simulink model "main_SEPETC"  (R2021a)
settings: Solver=VariableStepAuto  StartTime=0.0  StopTime=10  RelTol=1e-3
InitFcn:
  | run('Parameter.m')
values from neighbouring files (symbols this model uses):
  cp = 1    [Parameter.m]
  cv = 5    [Parameter.m]
  cw = 5    [Parameter.m]
  fref = 60    [Parameter.m]
  Lc1 = 0.35e-3    (= 0.00035)    [Parameter.m]
  Lc2 = 0.35e-3    (= 0.00035)    [Parameter.m]
  Lc3 = 0.35e-3    (= 0.00035)    [Parameter.m]
  Lc4 = 0.35e-3    (= 0.00035)    [Parameter.m]
  Lt12 = 318e-6    (= 0.000318)    [Parameter.m]
  Lt23 = 1847e-6    (= 0.001847)    [Parameter.m]
  Lt34 = 318e-6    (= 0.000318)    [Parameter.m]
  Mp1 = 9.4e-5    (= 9.4e-05)    [Parameter.m]
  Mp2 = 9.4e-5    (= 9.4e-05)    [Parameter.m]
  Mp3 = 12.5e-5    (= 0.000125)    [Parameter.m]
  Mp4 = 12.5e-5    (= 0.000125)    [Parameter.m]
  Nq1 = 1.3e-3    (= 0.0013)    [Parameter.m]
  Nq2 = 1.3e-3    (= 0.0013)    [Parameter.m]
  Nq3 = 1.5e-3    (= 0.0015)    [Parameter.m]
  Nq4 = 1.5e-3    (= 0.0015)    [Parameter.m]
  Rc1 = 0.03    [Parameter.m]
  Rc2 = 0.03    [Parameter.m]
  Rc3 = 0.03    [Parameter.m]
  Rc4 = 0.03    [Parameter.m]
  Rt12 = 0.23    [Parameter.m]
  Rt23 = 0.35    [Parameter.m]
  Rt34 = 0.23    [Parameter.m]
  t2 = 1    [Parameter.m]    (also in wvp_SEPETC.m)
  t3 = 10    [Parameter.m]
  t4 = 20    [Parameter.m]    (also in wvp_SEPETC.m = 21)
  t5 = 35    [Parameter.m]    (also in wvp_SEPETC.m = 33)
  t6 = 40    [Parameter.m]    (also in wvp_SEPETC.m = 35)
  Uo = 220*sqrt(2)    [Parameter.m]
  vref = 380    [Parameter.m]
  wc = 31.4    [Parameter.m]
  wref = 2*pi*fref    (= 376.991118431)    [Parameter.m]
undefined symbols (not defined in the file or in its folder): gcbh, sps_rtmsupport
libraries: spsControlledVoltageSourceLib x12, spsAlphaBetaZerotodq0Lib x12, eeGeneralControl x8, spsThreePhaseSeriesRLCBranchLib x7, spsGroundLib x4, spsThreePhaseVIMeasurementLib x4, spsThreePhaseBreakerLib x4, spsPLL3phLib x4, spsThreePhaseSeriesRLCLoadLib x3, spspowerguiLib x1
(part 3 of 3)

== system main_SEPETC/controller 1/primary 1/(P) abc to dq2 ==
  abc : Inport  PortDimensions=3
  wt : Inport  Port=2  PortDimensions=1
  Alpha-Beta-Zero to dq0 : spsAlphaBetaZerotodq0Lib/Alpha-Beta-Zero to dq0  Alignment=90 degrees behind phase A axis
      settings: SourceProductBaseCode=PS
  abc to Alpha-Beta-Zero : Subsystem  AncestorBlock=powerlib_meascontrol/Transformations/abc to Alpha-Beta-Zero  DialogController=POWERSYS.PowerSysDialog  LoadFcn=sps_rtmsupport('LoadFcn', gcbh);  StartFcn=sps_rtmsupport('StartFcn', gcbh);  StopFcn=sps_rtmsupport('StopFcn', gcbh);  mask(abc to Alpha-Beta-Zero Transformation){}
      mask help: Perform a Clarke transformation from a three-phase (abc) signal to a alpha-beta-zero stationary reference frame.
      settings: CopyFcn=sps_rtmsupport('CopyFcn', gcbh);  DeleteFcn=sps_rtmsupport('DeleteFcn', gcbh);  UndoDeleteFcn=sps_rtmsupport('UndoDeleteFcn', gcbh);  ModelCloseFcn=sps_rtmsupport('ModelCloseFcn', gcbh);  PreSaveFcn=sps_rtmsupport('PreSaveFcn', gcbh);  PostSaveFcn=sps_rtmsupport('PostSaveFcn', gcbh);  NameChangeFcn=sps_rtmsupport('NameChangeFcn', gcbh);  PreCopyFcn=sps_rtmsupport('PreCopyFcn', gcbh);  OpenFcn=sps_rtmsupport('OpenFcn', gcbh, []);  CloseFcn=sps_rtmsupport('CloseFcn', gcbh);  PreDeleteFcn=sps_rtmsupport('PreDeleteFcn', gcbh);
      mask Help: helpview(psbhelp);
      mask Display:
      | plot([0 1], [0,1])
      | text(0.15,0.7,'abc')
      | text(0.55, 0.3,'\alpha\beta0','texmode','on')
  dq0 : Outport  VectorParamsAs1DForOutWhenUnconnected=off
  wires:
  wt/1 -> Alpha-Beta-Zero to dq0/2
  abc/1 -> abc to Alpha-Beta-Zero/1(abc)
  Alpha-Beta-Zero to dq0/1 -> dq0/1
  abc to Alpha-Beta-Zero/1(al_be_0) -> Alpha-Beta-Zero to dq0/1

== system main_SEPETC/controller 2/(P) abc to dq2/abc to Alpha-Beta-Zero ==
  abc : Inport  PortDimensions=3
  Gain1 : Gain  Gain=sqrt(2/3)  SaturateOnIntegerOverflow=on  OutDataTypeStr=Inherit: Same as input  ParamDataTypeStr=Inherit: Same as input
  Gain3 : Gain  Gain="[ 1   -1/2   -1/2; 0   sqrt(3)/2   -sqrt(3)/2; 1/sqrt(2)  1/sqrt(2)  1/sqrt(2) ]"  Multiplication=Matrix(K*u) (u vector)  SaturateOnIntegerOverflow=on  OutDataTypeStr=Inherit: Same as input  ParamDataTypeStr=Inherit: Same as input
  al_be_0 : Outport  VectorParamsAs1DForOutWhenUnconnected=off
  wires:
  abc/1 -> Gain3/1
  Gain3/1 -> Gain1/1
  Gain1/1 -> al_be_0/1

== system main_SEPETC/controller 2/primary 1/(P) abc to dq1 ==
  abc : Inport  PortDimensions=3
  wt : Inport  Port=2  PortDimensions=1
  Alpha-Beta-Zero to dq0 : spsAlphaBetaZerotodq0Lib/Alpha-Beta-Zero to dq0  Alignment=90 degrees behind phase A axis
      settings: SourceProductBaseCode=PS
  abc to Alpha-Beta-Zero : Subsystem  AncestorBlock=powerlib_meascontrol/Transformations/abc to Alpha-Beta-Zero  DialogController=POWERSYS.PowerSysDialog  LoadFcn=sps_rtmsupport('LoadFcn', gcbh);  StartFcn=sps_rtmsupport('StartFcn', gcbh);  StopFcn=sps_rtmsupport('StopFcn', gcbh);  mask(abc to Alpha-Beta-Zero Transformation){}
      mask help: Perform a Clarke transformation from a three-phase (abc) signal to a alpha-beta-zero stationary reference frame.
      settings: CopyFcn=sps_rtmsupport('CopyFcn', gcbh);  DeleteFcn=sps_rtmsupport('DeleteFcn', gcbh);  UndoDeleteFcn=sps_rtmsupport('UndoDeleteFcn', gcbh);  ModelCloseFcn=sps_rtmsupport('ModelCloseFcn', gcbh);  PreSaveFcn=sps_rtmsupport('PreSaveFcn', gcbh);  PostSaveFcn=sps_rtmsupport('PostSaveFcn', gcbh);  NameChangeFcn=sps_rtmsupport('NameChangeFcn', gcbh);  PreCopyFcn=sps_rtmsupport('PreCopyFcn', gcbh);  OpenFcn=sps_rtmsupport('OpenFcn', gcbh, []);  CloseFcn=sps_rtmsupport('CloseFcn', gcbh);  PreDeleteFcn=sps_rtmsupport('PreDeleteFcn', gcbh);
      mask Help: helpview(psbhelp);
      mask Display:
      | plot([0 1], [0,1])
      | text(0.15,0.7,'abc')
      | text(0.55, 0.3,'\alpha\beta0','texmode','on')
  dq0 : Outport  VectorParamsAs1DForOutWhenUnconnected=off
  wires:
  wt/1 -> Alpha-Beta-Zero to dq0/2
  abc/1 -> abc to Alpha-Beta-Zero/1(abc)
  Alpha-Beta-Zero to dq0/1 -> dq0/1
  abc to Alpha-Beta-Zero/1(al_be_0) -> Alpha-Beta-Zero to dq0/1

== system main_SEPETC/controller 2/primary 1/(P) abc to dq2 ==
  abc : Inport  PortDimensions=3
  wt : Inport  Port=2  PortDimensions=1
  Alpha-Beta-Zero to dq0 : spsAlphaBetaZerotodq0Lib/Alpha-Beta-Zero to dq0  Alignment=90 degrees behind phase A axis
      settings: SourceProductBaseCode=PS
  abc to Alpha-Beta-Zero : Subsystem  AncestorBlock=powerlib_meascontrol/Transformations/abc to Alpha-Beta-Zero  DialogController=POWERSYS.PowerSysDialog  LoadFcn=sps_rtmsupport('LoadFcn', gcbh);  StartFcn=sps_rtmsupport('StartFcn', gcbh);  StopFcn=sps_rtmsupport('StopFcn', gcbh);  mask(abc to Alpha-Beta-Zero Transformation){}
      mask help: Perform a Clarke transformation from a three-phase (abc) signal to a alpha-beta-zero stationary reference frame.
      settings: CopyFcn=sps_rtmsupport('CopyFcn', gcbh);  DeleteFcn=sps_rtmsupport('DeleteFcn', gcbh);  UndoDeleteFcn=sps_rtmsupport('UndoDeleteFcn', gcbh);  ModelCloseFcn=sps_rtmsupport('ModelCloseFcn', gcbh);  PreSaveFcn=sps_rtmsupport('PreSaveFcn', gcbh);  PostSaveFcn=sps_rtmsupport('PostSaveFcn', gcbh);  NameChangeFcn=sps_rtmsupport('NameChangeFcn', gcbh);  PreCopyFcn=sps_rtmsupport('PreCopyFcn', gcbh);  OpenFcn=sps_rtmsupport('OpenFcn', gcbh, []);  CloseFcn=sps_rtmsupport('CloseFcn', gcbh);  PreDeleteFcn=sps_rtmsupport('PreDeleteFcn', gcbh);
      mask Help: helpview(psbhelp);
      mask Display:
      | plot([0 1], [0,1])
      | text(0.15,0.7,'abc')
      | text(0.55, 0.3,'\alpha\beta0','texmode','on')
  dq0 : Outport  VectorParamsAs1DForOutWhenUnconnected=off
  wires:
  wt/1 -> Alpha-Beta-Zero to dq0/2
  abc/1 -> abc to Alpha-Beta-Zero/1(abc)
  Alpha-Beta-Zero to dq0/1 -> dq0/1
  abc to Alpha-Beta-Zero/1(al_be_0) -> Alpha-Beta-Zero to dq0/1

== system main_SEPETC/controller 3/(P) abc to dq2/abc to Alpha-Beta-Zero ==
  abc : Inport  PortDimensions=3
  Gain1 : Gain  Gain=sqrt(2/3)  SaturateOnIntegerOverflow=on  OutDataTypeStr=Inherit: Same as input  ParamDataTypeStr=Inherit: Same as input
  Gain3 : Gain  Gain="[ 1   -1/2   -1/2; 0   sqrt(3)/2   -sqrt(3)/2; 1/sqrt(2)  1/sqrt(2)  1/sqrt(2) ]"  Multiplication=Matrix(K*u) (u vector)  SaturateOnIntegerOverflow=on  OutDataTypeStr=Inherit: Same as input  ParamDataTypeStr=Inherit: Same as input
  al_be_0 : Outport  VectorParamsAs1DForOutWhenUnconnected=off
  wires:
  abc/1 -> Gain3/1
  Gain3/1 -> Gain1/1
  Gain1/1 -> al_be_0/1

== system main_SEPETC/controller 3/primary 3/(P) abc to dq1 ==
  abc : Inport  PortDimensions=3
  wt : Inport  Port=2  PortDimensions=1
  Alpha-Beta-Zero to dq0 : spsAlphaBetaZerotodq0Lib/Alpha-Beta-Zero to dq0  Alignment=90 degrees behind phase A axis
      settings: SourceProductBaseCode=PS
  abc to Alpha-Beta-Zero : Subsystem  AncestorBlock=powerlib_meascontrol/Transformations/abc to Alpha-Beta-Zero  DialogController=POWERSYS.PowerSysDialog  LoadFcn=sps_rtmsupport('LoadFcn', gcbh);  StartFcn=sps_rtmsupport('StartFcn', gcbh);  StopFcn=sps_rtmsupport('StopFcn', gcbh);  mask(abc to Alpha-Beta-Zero Transformation){}
      mask help: Perform a Clarke transformation from a three-phase (abc) signal to a alpha-beta-zero stationary reference frame.
      settings: CopyFcn=sps_rtmsupport('CopyFcn', gcbh);  DeleteFcn=sps_rtmsupport('DeleteFcn', gcbh);  UndoDeleteFcn=sps_rtmsupport('UndoDeleteFcn', gcbh);  ModelCloseFcn=sps_rtmsupport('ModelCloseFcn', gcbh);  PreSaveFcn=sps_rtmsupport('PreSaveFcn', gcbh);  PostSaveFcn=sps_rtmsupport('PostSaveFcn', gcbh);  NameChangeFcn=sps_rtmsupport('NameChangeFcn', gcbh);  PreCopyFcn=sps_rtmsupport('PreCopyFcn', gcbh);  OpenFcn=sps_rtmsupport('OpenFcn', gcbh, []);  CloseFcn=sps_rtmsupport('CloseFcn', gcbh);  PreDeleteFcn=sps_rtmsupport('PreDeleteFcn', gcbh);
      mask Help: helpview(psbhelp);
      mask Display:
      | plot([0 1], [0,1])
      | text(0.15,0.7,'abc')
      | text(0.55, 0.3,'\alpha\beta0','texmode','on')
  dq0 : Outport  VectorParamsAs1DForOutWhenUnconnected=off
  wires:
  wt/1 -> Alpha-Beta-Zero to dq0/2
  abc/1 -> abc to Alpha-Beta-Zero/1(abc)
  Alpha-Beta-Zero to dq0/1 -> dq0/1
  abc to Alpha-Beta-Zero/1(al_be_0) -> Alpha-Beta-Zero to dq0/1

== system main_SEPETC/controller 3/primary 3/(P) abc to dq2 ==
  abc : Inport  PortDimensions=3
  wt : Inport  Port=2  PortDimensions=1
  Alpha-Beta-Zero to dq0 : spsAlphaBetaZerotodq0Lib/Alpha-Beta-Zero to dq0  Alignment=90 degrees behind phase A axis
      settings: SourceProductBaseCode=PS
  abc to Alpha-Beta-Zero : Subsystem  AncestorBlock=powerlib_meascontrol/Transformations/abc to Alpha-Beta-Zero  DialogController=POWERSYS.PowerSysDialog  LoadFcn=sps_rtmsupport('LoadFcn', gcbh);  StartFcn=sps_rtmsupport('StartFcn', gcbh);  StopFcn=sps_rtmsupport('StopFcn', gcbh);  mask(abc to Alpha-Beta-Zero Transformation){}
      mask help: Perform a Clarke transformation from a three-phase (abc) signal to a alpha-beta-zero stationary reference frame.
      settings: CopyFcn=sps_rtmsupport('CopyFcn', gcbh);  DeleteFcn=sps_rtmsupport('DeleteFcn', gcbh);  UndoDeleteFcn=sps_rtmsupport('UndoDeleteFcn', gcbh);  ModelCloseFcn=sps_rtmsupport('ModelCloseFcn', gcbh);  PreSaveFcn=sps_rtmsupport('PreSaveFcn', gcbh);  PostSaveFcn=sps_rtmsupport('PostSaveFcn', gcbh);  NameChangeFcn=sps_rtmsupport('NameChangeFcn', gcbh);  PreCopyFcn=sps_rtmsupport('PreCopyFcn', gcbh);  OpenFcn=sps_rtmsupport('OpenFcn', gcbh, []);  CloseFcn=sps_rtmsupport('CloseFcn', gcbh);  PreDeleteFcn=sps_rtmsupport('PreDeleteFcn', gcbh);
      mask Help: helpview(psbhelp);
      mask Display:
      | plot([0 1], [0,1])
      | text(0.15,0.7,'abc')
      | text(0.55, 0.3,'\alpha\beta0','texmode','on')
  dq0 : Outport  VectorParamsAs1DForOutWhenUnconnected=off
  wires:
  wt/1 -> Alpha-Beta-Zero to dq0/2
  abc/1 -> abc to Alpha-Beta-Zero/1(abc)
  Alpha-Beta-Zero to dq0/1 -> dq0/1
  abc to Alpha-Beta-Zero/1(al_be_0) -> Alpha-Beta-Zero to dq0/1

== system main_SEPETC/controller 3/v_secondary 3/Subsystem2 ==
  In1 : Inport
  Constant : Constant  Value=0
  Switch : Switch  Criteria=u2 > Threshold
  Out1 : Outport
  wires:
  [t] -> Switch/2
  Switch/1 -> Out1/1
  Constant/1 -> Switch/3
  In1/1 -> Switch/1

== system main_SEPETC/controller 3/w_secondary 3/Subsystem2 ==
  In1 : Inport
  Constant : Constant  Value=0
  Switch : Switch  Criteria=u2 > Threshold
  Out1 : Outport
  wires:
  [t] -> Switch/2
  Switch/1 -> Out1/1
  Constant/1 -> Switch/3
  In1/1 -> Switch/1

== system main_SEPETC/controller 4/(P) abc to dq2/abc to Alpha-Beta-Zero ==
  abc : Inport  PortDimensions=3
  Gain1 : Gain  Gain=sqrt(2/3)  SaturateOnIntegerOverflow=on  OutDataTypeStr=Inherit: Same as input  ParamDataTypeStr=Inherit: Same as input
  Gain3 : Gain  Gain="[ 1   -1/2   -1/2; 0   sqrt(3)/2   -sqrt(3)/2; 1/sqrt(2)  1/sqrt(2)  1/sqrt(2) ]"  Multiplication=Matrix(K*u) (u vector)  SaturateOnIntegerOverflow=on  OutDataTypeStr=Inherit: Same as input  ParamDataTypeStr=Inherit: Same as input
  al_be_0 : Outport  VectorParamsAs1DForOutWhenUnconnected=off
  wires:
  abc/1 -> Gain3/1
  Gain3/1 -> Gain1/1
  Gain1/1 -> al_be_0/1

== system main_SEPETC/controller 4/primary 3/Subsystem1 ==
  note: D-Q变换
  Vo1 : Inport
  wt : Inport  Port=2
  io1 : Inport  Port=3
  (P) abc to dq1 : Subsystem  AncestorBlock=powerlib_meascontrol/Transformations/abc to dq0  DialogController=POWERSYS.PowerSysDialog  LoadFcn=sps_rtmsupport('LoadFcn', gcbh);  StartFcn=sps_rtmsupport('StartFcn', gcbh);  StopFcn=sps_rtmsupport('StopFcn', gcbh);  mask(abc to dq0 Transformation){Alignment=90 degrees behind phase A axis}
      mask prompts: Alignment "Rotating frame alignment at wt=0:"
      mask help:
      | Perform a Park transformation from a three-phase (abc) signal to a dq0 rotating reference frame. Angular position of the rotating frame is given by input wt (rad).
      |
      | When the rotating frame alignment at wt=0 is 90 degrees behind phase A axis, a positive-sequence signal with Mag=1 & Phase=0 degrees yields the following dq values: d=1, q=0.
      mask init:
      | str=cat(2,gcb,'/Alpha-Beta-Zero to dq0');
      | if Alignment==1
      |     set_param(str,'Alignment','Aligned with phase A axis');
      | else
      |     set_param(str,'Alignment','90 degrees behind phase A axis');
      | end
      settings: CopyFcn=sps_rtmsupport('CopyFcn', gcbh);  DeleteFcn=sps_rtmsupport('DeleteFcn', gcbh);  UndoDeleteFcn=sps_rtmsupport('UndoDeleteFcn', gcbh);  ModelCloseFcn=sps_rtmsupport('ModelCloseFcn', gcbh);  PreSaveFcn=sps_rtmsupport('PreSaveFcn', gcbh);  PostSaveFcn=sps_rtmsupport('PostSaveFcn', gcbh);  NameChangeFcn=sps_rtmsupport('NameChangeFcn', gcbh);  PreCopyFcn=sps_rtmsupport('PreCopyFcn', gcbh);  OpenFcn=sps_rtmsupport('OpenFcn', gcbh, [1]);  CloseFcn=sps_rtmsupport('CloseFcn', gcbh);  PreDeleteFcn=sps_rtmsupport('PreDeleteFcn', gcbh);
      mask Help: helpview(psbhelp);
      mask TypeOptions Alignment: Aligned with phase A axis | 90 degrees behind phase A axis
      mask Display:
      | plot([0 1], [0,1])
      | port_label('input', 1, 'abc')
      | port_label('input', 2, 'wt')
      | port_label('output', 1, 'dq0')
  (P) abc to dq2 : Subsystem  AncestorBlock=powerlib_meascontrol/Transformations/abc to dq0  DialogController=POWERSYS.PowerSysDialog  LoadFcn=sps_rtmsupport('LoadFcn', gcbh);  StartFcn=sps_rtmsupport('StartFcn', gcbh);  StopFcn=sps_rtmsupport('StopFcn', gcbh);  mask(abc to dq0 Transformation){Alignment=90 degrees behind phase A axis}
      mask prompts: Alignment "Rotating frame alignment at wt=0:"
      mask help:
      | Perform a Park transformation from a three-phase (abc) signal to a dq0 rotating reference frame. Angular position of the rotating frame is given by input wt (rad).
      |
      | When the rotating frame alignment at wt=0 is 90 degrees behind phase A axis, a positive-sequence signal with Mag=1 & Phase=0 degrees yields the following dq values: d=1, q=0.
      mask init:
      | str=cat(2,gcb,'/Alpha-Beta-Zero to dq0');
      | if Alignment==1
      |     set_param(str,'Alignment','Aligned with phase A axis');
      | else
      |     set_param(str,'Alignment','90 degrees behind phase A axis');
      | end
      settings: CopyFcn=sps_rtmsupport('CopyFcn', gcbh);  DeleteFcn=sps_rtmsupport('DeleteFcn', gcbh);  UndoDeleteFcn=sps_rtmsupport('UndoDeleteFcn', gcbh);  ModelCloseFcn=sps_rtmsupport('ModelCloseFcn', gcbh);  PreSaveFcn=sps_rtmsupport('PreSaveFcn', gcbh);  PostSaveFcn=sps_rtmsupport('PostSaveFcn', gcbh);  NameChangeFcn=sps_rtmsupport('NameChangeFcn', gcbh);  PreCopyFcn=sps_rtmsupport('PreCopyFcn', gcbh);  OpenFcn=sps_rtmsupport('OpenFcn', gcbh, [1]);  CloseFcn=sps_rtmsupport('CloseFcn', gcbh);  PreDeleteFcn=sps_rtmsupport('PreDeleteFcn', gcbh);
      mask Help: helpview(psbhelp);
      mask TypeOptions Alignment: Aligned with phase A axis | 90 degrees behind phase A axis
      mask Display:
      | plot([0 1], [0,1])
      | port_label('input', 1, 'abc')
      | port_label('input', 2, 'wt')
      | port_label('output', 1, 'dq0')
  Demux : Demux  Outputs=2
  Demux1 : Demux  Outputs=2
  Gain : Gain
  Gain1 : Gain
  Product{,1..3} (4 alike) : Product
  Selector : Selector  InputPortWidth=3  IndexOptions=Index vector (dialog)  Indices=[1 2]  OutputSizes=1
  Selector1 : Selector  InputPortWidth=3  IndexOptions=Index vector (dialog)  Indices=[1 2]  OutputSizes=1
  Sum2 : Sum  Inputs=|++
  Sum3 : Sum  Inputs=|-+
  p' : Outport
  q' : Outport  Port=2
  wires:
  Selector/1 -> Demux/1
  Demux/2 -> Product1/1, Product3/1  "voqi"
  Selector1/1 -> Demux1/1
  wt/1 -> (P) abc to dq1/2(wt), (P) abc to dq2/2(wt)
  Demux/1 -> Product2/1, Product/1  "vodi"
  (P) abc to dq2/1(dq0) -> Selector/1
  Demux1/1 -> Product3/2, Product/2  "iodi"
  (P) abc to dq1/1(dq0) -> Selector1/1
  Product3/1 -> Sum3/2
  Product2/1 -> Sum3/1
  Demux1/2 -> Product1/2, Product2/2  "ioqi"
  Product1/1 -> Sum2/2
  Product/1 -> Sum2/1
  io1/1 -> (P) abc to dq1/1(abc)
  Vo1/1 -> (P) abc to dq2/1(abc)
  Sum2/1 -> Gain/1
  Sum3/1 -> Gain1/1
  Gain1/1 -> q'/1
  Gain/1 -> p'/1

== system main_SEPETC/active power sharing SE-PETC /EState_1/x1_o2/Subsystem1 ==
  In1 : Inport
  Constant : Constant  Value=0
  Switch : Switch  Criteria=u2 > Threshold
  Out1 : Outport
  wires:
  [t] -> Switch/2
  Switch/1 -> Out1/1
  Constant/1 -> Switch/3
  In1/1 -> Switch/1

== system main_SEPETC/active power sharing SE-PETC /EState_1/x1_o4/Subsystem4 ==
  In1 : Inport
  Constant : Constant  Value=0
  Switch : Switch  Criteria=u2 > Threshold
  Out1 : Outport
  wires:
  [t] -> Switch/2
  Switch/1 -> Out1/1
  Constant/1 -> Switch/3
  In1/1 -> Switch/1

== system main_SEPETC/active power sharing SE-PETC /EState_2/x2_o2/Subsystem1 ==
  In1 : Inport
  Constant : Constant  Value=0
  Switch : Switch  Criteria=u2 > Threshold
  Out1 : Outport
  wires:
  [t] -> Switch/2
  Switch/1 -> Out1/1
  In1/1 -> Switch/1
  Constant/1 -> Switch/3

== system main_SEPETC/active power sharing SE-PETC /EState_2/x2_o3/Subsystem1 ==
  In1 : Inport
  Constant : Constant  Value=0
  Switch : Switch  Criteria=u2 > Threshold
  Out1 : Outport
  wires:
  [t] -> Switch/2
  Switch/1 -> Out1/1
  Constant/1 -> Switch/3
  In1/1 -> Switch/1

== system main_SEPETC/active power sharing SE-PETC /EState_2/x2_o3/Subsystem2 ==
  In1 : Inport
  Constant : Constant  Value=0
  Switch : Switch  Criteria=u2 > Threshold
  Out1 : Outport
  wires:
  [t] -> Switch/2
  Switch/1 -> Out1/1
  Constant/1 -> Switch/3
  In1/1 -> Switch/1

== system main_SEPETC/active power sharing SE-PETC /EState_2/x2_o3/Subsystem3 ==
  In1 : Inport
  Constant : Constant  Value=0
  Switch : Switch  Criteria=u2 > Threshold
  Out1 : Outport
  wires:
  [t] -> Switch/2
  Switch/1 -> Out1/1
  Constant/1 -> Switch/3
  In1/1 -> Switch/1

== system main_SEPETC/active power sharing SE-PETC /EState_2/x2_o3/Subsystem4 ==
  In1 : Inport
  Constant : Constant  Value=0
  Switch : Switch  Criteria=u2 > Threshold
  Out1 : Outport
  wires:
  [t] -> Switch/2
  Switch/1 -> Out1/1
  Constant/1 -> Switch/3
  In1/1 -> Switch/1

== system main_SEPETC/active power sharing SE-PETC /EState_3/x3_o2/Subsystem1 ==
  In1 : Inport
  Constant : Constant  Value=0
  Switch : Switch  Criteria=u2 > Threshold
  Out1 : Outport
  wires:
  [t] -> Switch/2
  Switch/1 -> Out1/1
  Constant/1 -> Switch/3
  In1/1 -> Switch/1

== system main_SEPETC/active power sharing SE-PETC /EState_3/x3_o2/Subsystem2 ==
  In1 : Inport
  Constant : Constant  Value=0
  Switch : Switch  Criteria=u2 > Threshold
  Out1 : Outport
  wires:
  [t] -> Switch/2
  Switch/1 -> Out1/1
  Constant/1 -> Switch/3
  In1/1 -> Switch/1

== system main_SEPETC/active power sharing SE-PETC /EState_3/x3_o2/Subsystem3 ==
  In1 : Inport
  Constant : Constant  Value=0
  Switch : Switch  Criteria=u2 > Threshold
  Out1 : Outport
  wires:
  [t] -> Switch/2
  Switch/1 -> Out1/1
  Constant/1 -> Switch/3
  In1/1 -> Switch/1

== system main_SEPETC/active power sharing SE-PETC /EState_3/x3_o2/Subsystem4 ==
  In1 : Inport
  Constant : Constant  Value=0
  Switch : Switch  Criteria=u2 > Threshold
  Out1 : Outport
  wires:
  [t] -> Switch/2
  Switch/1 -> Out1/1
  Constant/1 -> Switch/3
  In1/1 -> Switch/1

== system main_SEPETC/active power sharing SE-PETC /EState_3/x3_o3/Subsystem1 ==
  In1 : Inport
  Constant : Constant  Value=0
  Switch : Switch  Criteria=u2 > Threshold
  Out1 : Outport
  wires:
  [t] -> Switch/2
  Switch/1 -> Out1/1
  Constant/1 -> Switch/3
  In1/1 -> Switch/1

== system main_SEPETC/active power sharing SE-PETC /EState_3/x3_o3/Subsystem2 ==
  In1 : Inport
  Constant : Constant  Value=0
  Switch : Switch  Criteria=u2 > Threshold
  Out1 : Outport
  wires:
  [t] -> Switch/2
  Switch/1 -> Out1/1
  Constant/1 -> Switch/3
  In1/1 -> Switch/1

== system main_SEPETC/active power sharing SE-PETC /EState_3/x3_o3/Subsystem3 ==
  In1 : Inport
  Constant : Constant  Value=0
  Switch : Switch  Criteria=u2 > Threshold
  Out1 : Outport
  wires:
  [t] -> Switch/2
  Switch/1 -> Out1/1
  Constant/1 -> Switch/3
  In1/1 -> Switch/1

== system main_SEPETC/active power sharing SE-PETC /EState_3/x3_o3/Subsystem4 ==
  In1 : Inport
  Constant : Constant  Value=0
  Switch : Switch  Criteria=u2 > Threshold
  Out1 : Outport
  wires:
  [t] -> Switch/2
  Switch/1 -> Out1/1
  Constant/1 -> Switch/3
  In1/1 -> Switch/1

== system main_SEPETC/active power sharing SE-PETC /EState_3/x3_o4/Subsystem1 ==
  In1 : Inport
  Constant : Constant  Value=0
  Switch : Switch  Criteria=u2 > Threshold
  Out1 : Outport
  wires:
  [t] -> Switch/2
  Switch/1 -> Out1/1
  Constant/1 -> Switch/3
  In1/1 -> Switch/1

== system main_SEPETC/active power sharing SE-PETC /EState_3/x3_o4/Subsystem2 ==
  In1 : Inport
  Constant : Constant  Value=0
  Switch : Switch  Criteria=u2 > Threshold
  Out1 : Outport
  wires:
  [t] -> Switch/2
  Switch/1 -> Out1/1
  Constant/1 -> Switch/3
  In1/1 -> Switch/1

== system main_SEPETC/active power sharing SE-PETC /EState_3/x3_o4/Subsystem3 ==
  In1 : Inport
  Constant : Constant  Value=0
  Switch : Switch  Criteria=u2 > Threshold
  Out1 : Outport
  wires:
  [t] -> Switch/2
  Switch/1 -> Out1/1
  Constant/1 -> Switch/3
  In1/1 -> Switch/1

== system main_SEPETC/active power sharing SE-PETC /EState_3/x3_o4/Subsystem4 ==
  In1 : Inport
  Constant : Constant  Value=0
  Switch : Switch  Criteria=u2 > Threshold
  x3_o4 : Outport
  wires:
  [t] -> Switch/2
  Switch/1 -> x3_o4/1
  Constant/1 -> Switch/3
  In1/1 -> Switch/1

== system main_SEPETC/active power sharing SE-PETC /EState_4/x4_o3/Subsystem1 ==
  In1 : Inport
  Constant : Constant  Value=0
  Switch : Switch  Criteria=u2 > Threshold
  Out1 : Outport
  wires:
  [t] -> Switch/2
  Switch/1 -> Out1/1
  Constant/1 -> Switch/3
  In1/1 -> Switch/1

== system main_SEPETC/active power sharing SE-PETC /EState_4/x4_o3/Subsystem2 ==
  In1 : Inport
  Constant : Constant  Value=0
  Switch : Switch  Criteria=u2 > Threshold
  Out1 : Outport
  wires:
  [t] -> Switch/2
  Switch/1 -> Out1/1
  Constant/1 -> Switch/3
  In1/1 -> Switch/1

== system main_SEPETC/active power sharing SE-PETC /EState_4/x4_o3/Subsystem3 ==
  In1 : Inport
  Constant : Constant  Value=0
  Switch : Switch  Criteria=u2 > Threshold
  Out1 : Outport
  wires:
  [t] -> Switch/2
  Switch/1 -> Out1/1
  Constant/1 -> Switch/3
  In1/1 -> Switch/1

== system main_SEPETC/active power sharing SE-PETC /EState_4/x4_o3/Subsystem4 ==
  In1 : Inport
  Constant : Constant  Value=0
  Switch : Switch  Criteria=u2 > Threshold
  Out1 : Outport
  wires:
  [t] -> Switch/2
  Switch/1 -> Out1/1
  Constant/1 -> Switch/3
  In1/1 -> Switch/1

== system main_SEPETC/active power sharing SE-PETC /EState_4/x4_o4/Subsystem1 ==
  In1 : Inport
  Constant : Constant  Value=0
  Switch : Switch  Criteria=u2 > Threshold
  Out1 : Outport
  wires:
  [t] -> Switch/2
  Switch/1 -> Out1/1
  Constant/1 -> Switch/3
  In1/1 -> Switch/1

== system main_SEPETC/active power sharing SE-PETC 1/EState_1/x1_o2/Subsystem1 ==
  In1 : Inport
  Constant : Constant  Value=0
  Switch : Switch  Criteria=u2 > Threshold
  Out1 : Outport
  wires:
  [t] -> Switch/2
  Switch/1 -> Out1/1
  Constant/1 -> Switch/3
  In1/1 -> Switch/1

== system main_SEPETC/active power sharing SE-PETC 1/EState_1/x1_o4/Subsystem4 ==
  In1 : Inport
  Constant : Constant  Value=0
  Switch : Switch  Criteria=u2 > Threshold
  Out1 : Outport
  wires:
  [t] -> Switch/2
  Switch/1 -> Out1/1
  Constant/1 -> Switch/3
  In1/1 -> Switch/1

== system main_SEPETC/active power sharing SE-PETC 1/EState_2/x2_o2/Subsystem1 ==
  In1 : Inport
  Constant : Constant  Value=0
  Switch : Switch  Criteria=u2 > Threshold
  Out1 : Outport
  wires:
  [t] -> Switch/2
  Switch/1 -> Out1/1
  In1/1 -> Switch/1
  Constant/1 -> Switch/3

== system main_SEPETC/active power sharing SE-PETC 1/EState_2/x2_o3/Subsystem1 ==
  In1 : Inport
  Constant : Constant  Value=0
  Switch : Switch  Criteria=u2 > Threshold
  Out1 : Outport
  wires:
  [t] -> Switch/2
  Switch/1 -> Out1/1
  Constant/1 -> Switch/3
  In1/1 -> Switch/1

== system main_SEPETC/active power sharing SE-PETC 1/EState_2/x2_o3/Subsystem2 ==
  In1 : Inport
  Constant : Constant  Value=0
  Switch : Switch  Criteria=u2 > Threshold
  Out1 : Outport
  wires:
  [t] -> Switch/2
  Switch/1 -> Out1/1
  Constant/1 -> Switch/3
  In1/1 -> Switch/1

== system main_SEPETC/active power sharing SE-PETC 1/EState_2/x2_o3/Subsystem3 ==
  In1 : Inport
  Constant : Constant  Value=0
  Switch : Switch  Criteria=u2 > Threshold
  Out1 : Outport
  wires:
  [t] -> Switch/2
  Switch/1 -> Out1/1
  Constant/1 -> Switch/3
  In1/1 -> Switch/1

== system main_SEPETC/active power sharing SE-PETC 1/EState_2/x2_o3/Subsystem4 ==
  In1 : Inport
  Constant : Constant  Value=0
  Switch : Switch  Criteria=u2 > Threshold
  Out1 : Outport
  wires:
  [t] -> Switch/2
  Switch/1 -> Out1/1
  Constant/1 -> Switch/3
  In1/1 -> Switch/1

== system main_SEPETC/active power sharing SE-PETC 1/EState_3/x3_o2/Subsystem1 ==
  In1 : Inport
  Constant : Constant  Value=0
  Switch : Switch  Criteria=u2 > Threshold
  Out1 : Outport
  wires:
  [t] -> Switch/2
  Switch/1 -> Out1/1
  Constant/1 -> Switch/3
  In1/1 -> Switch/1

== system main_SEPETC/active power sharing SE-PETC 1/EState_3/x3_o2/Subsystem2 ==
  In1 : Inport
  Constant : Constant  Value=0
  Switch : Switch  Criteria=u2 > Threshold
  Out1 : Outport
  wires:
  [t] -> Switch/2
  Switch/1 -> Out1/1
  Constant/1 -> Switch/3
  In1/1 -> Switch/1

== system main_SEPETC/active power sharing SE-PETC 1/EState_3/x3_o2/Subsystem3 ==
  In1 : Inport
  Constant : Constant  Value=0
  Switch : Switch  Criteria=u2 > Threshold
  Out1 : Outport
  wires:
  [t] -> Switch/2
  Switch/1 -> Out1/1
  Constant/1 -> Switch/3
  In1/1 -> Switch/1

== system main_SEPETC/active power sharing SE-PETC 1/EState_3/x3_o2/Subsystem4 ==
  In1 : Inport
  Constant : Constant  Value=0
  Switch : Switch  Criteria=u2 > Threshold
  Out1 : Outport
  wires:
  [t] -> Switch/2
  Switch/1 -> Out1/1
  Constant/1 -> Switch/3
  In1/1 -> Switch/1

== system main_SEPETC/active power sharing SE-PETC 1/EState_3/x3_o3/Subsystem1 ==
  In1 : Inport
  Constant : Constant  Value=0
  Switch : Switch  Criteria=u2 > Threshold
  Out1 : Outport
  wires:
  [t] -> Switch/2
  Switch/1 -> Out1/1
  Constant/1 -> Switch/3
  In1/1 -> Switch/1

== system main_SEPETC/active power sharing SE-PETC 1/EState_3/x3_o3/Subsystem2 ==
  In1 : Inport
  Constant : Constant  Value=0
  Switch : Switch  Criteria=u2 > Threshold
  Out1 : Outport
  wires:
  [t] -> Switch/2
  Switch/1 -> Out1/1
  Constant/1 -> Switch/3
  In1/1 -> Switch/1

== system main_SEPETC/active power sharing SE-PETC 1/EState_3/x3_o3/Subsystem3 ==
  In1 : Inport
  Constant : Constant  Value=0
  Switch : Switch  Criteria=u2 > Threshold
  Out1 : Outport
  wires:
  [t] -> Switch/2
  Switch/1 -> Out1/1
  Constant/1 -> Switch/3
  In1/1 -> Switch/1

== system main_SEPETC/active power sharing SE-PETC 1/EState_3/x3_o3/Subsystem4 ==
  In1 : Inport
  Constant : Constant  Value=0
  Switch : Switch  Criteria=u2 > Threshold
  Out1 : Outport
  wires:
  [t] -> Switch/2
  Switch/1 -> Out1/1
  Constant/1 -> Switch/3
  In1/1 -> Switch/1

== system main_SEPETC/active power sharing SE-PETC 1/EState_3/x3_o4/Subsystem1 ==
  In1 : Inport
  Constant : Constant  Value=0
  Switch : Switch  Criteria=u2 > Threshold
  Out1 : Outport
  wires:
  [t] -> Switch/2
  Switch/1 -> Out1/1
  Constant/1 -> Switch/3
  In1/1 -> Switch/1

== system main_SEPETC/active power sharing SE-PETC 1/EState_3/x3_o4/Subsystem2 ==
  In1 : Inport
  Constant : Constant  Value=0
  Switch : Switch  Criteria=u2 > Threshold
  Out1 : Outport
  wires:
  [t] -> Switch/2
  Switch/1 -> Out1/1
  Constant/1 -> Switch/3
  In1/1 -> Switch/1

== system main_SEPETC/active power sharing SE-PETC 1/EState_3/x3_o4/Subsystem3 ==
  In1 : Inport
  Constant : Constant  Value=0
  Switch : Switch  Criteria=u2 > Threshold
  Out1 : Outport
  wires:
  [t] -> Switch/2
  Switch/1 -> Out1/1
  Constant/1 -> Switch/3
  In1/1 -> Switch/1

== system main_SEPETC/active power sharing SE-PETC 1/EState_3/x3_o4/Subsystem4 ==
  In1 : Inport
  Constant : Constant  Value=0
  Switch : Switch  Criteria=u2 > Threshold
  x3_o4 : Outport
  wires:
  [t] -> Switch/2
  Switch/1 -> x3_o4/1
  Constant/1 -> Switch/3
  In1/1 -> Switch/1

== system main_SEPETC/active power sharing SE-PETC 1/EState_4/x4_o3/Subsystem1 ==
  In1 : Inport
  Constant : Constant  Value=0
  Switch : Switch  Criteria=u2 > Threshold
  Out1 : Outport
  wires:
  [t] -> Switch/2
  Switch/1 -> Out1/1
  Constant/1 -> Switch/3
  In1/1 -> Switch/1

== system main_SEPETC/active power sharing SE-PETC 1/EState_4/x4_o3/Subsystem2 ==
  In1 : Inport
  Constant : Constant  Value=0
  Switch : Switch  Criteria=u2 > Threshold
  Out1 : Outport
  wires:
  [t] -> Switch/2
  Switch/1 -> Out1/1
  Constant/1 -> Switch/3
  In1/1 -> Switch/1

== system main_SEPETC/active power sharing SE-PETC 1/EState_4/x4_o3/Subsystem3 ==
  In1 : Inport
  Constant : Constant  Value=0
  Switch : Switch  Criteria=u2 > Threshold
  Out1 : Outport
  wires:
  [t] -> Switch/2
  Switch/1 -> Out1/1
  Constant/1 -> Switch/3
  In1/1 -> Switch/1

== system main_SEPETC/active power sharing SE-PETC 1/EState_4/x4_o3/Subsystem4 ==
  In1 : Inport
  Constant : Constant  Value=0
  Switch : Switch  Criteria=u2 > Threshold
  Out1 : Outport
  wires:
  [t] -> Switch/2
  Switch/1 -> Out1/1
  Constant/1 -> Switch/3
  In1/1 -> Switch/1

== system main_SEPETC/active power sharing SE-PETC 1/EState_4/x4_o4/Subsystem1 ==
  In1 : Inport
  Constant : Constant  Value=0
  Switch : Switch  Criteria=u2 > Threshold
  Out1 : Outport
  wires:
  [t] -> Switch/2
  Switch/1 -> Out1/1
  Constant/1 -> Switch/3
  In1/1 -> Switch/1

== system main_SEPETC/controller 1/primary 1/(P) abc to dq1/abc to Alpha-Beta-Zero ==
  abc : Inport  PortDimensions=3
  Gain1 : Gain  Gain=sqrt(2/3)  SaturateOnIntegerOverflow=on  OutDataTypeStr=Inherit: Same as input  ParamDataTypeStr=Inherit: Same as input
  Gain3 : Gain  Gain="[ 1   -1/2   -1/2; 0   sqrt(3)/2   -sqrt(3)/2; 1/sqrt(2)  1/sqrt(2)  1/sqrt(2) ]"  Multiplication=Matrix(K*u) (u vector)  SaturateOnIntegerOverflow=on  OutDataTypeStr=Inherit: Same as input  ParamDataTypeStr=Inherit: Same as input
  al_be_0 : Outport  VectorParamsAs1DForOutWhenUnconnected=off
  wires:
  abc/1 -> Gain3/1
  Gain3/1 -> Gain1/1
  Gain1/1 -> al_be_0/1

== system main_SEPETC/controller 1/primary 1/(P) abc to dq2/abc to Alpha-Beta-Zero ==
  abc : Inport  PortDimensions=3
  Gain1 : Gain  Gain=sqrt(2/3)  SaturateOnIntegerOverflow=on  OutDataTypeStr=Inherit: Same as input  ParamDataTypeStr=Inherit: Same as input
  Gain3 : Gain  Gain="[ 1   -1/2   -1/2; 0   sqrt(3)/2   -sqrt(3)/2; 1/sqrt(2)  1/sqrt(2)  1/sqrt(2) ]"  Multiplication=Matrix(K*u) (u vector)  SaturateOnIntegerOverflow=on  OutDataTypeStr=Inherit: Same as input  ParamDataTypeStr=Inherit: Same as input
  al_be_0 : Outport  VectorParamsAs1DForOutWhenUnconnected=off
  wires:
  abc/1 -> Gain3/1
  Gain3/1 -> Gain1/1
  Gain1/1 -> al_be_0/1

== system main_SEPETC/controller 2/primary 1/(P) abc to dq1/abc to Alpha-Beta-Zero ==
  abc : Inport  PortDimensions=3
  Gain1 : Gain  Gain=sqrt(2/3)  SaturateOnIntegerOverflow=on  OutDataTypeStr=Inherit: Same as input  ParamDataTypeStr=Inherit: Same as input
  Gain3 : Gain  Gain="[ 1   -1/2   -1/2; 0   sqrt(3)/2   -sqrt(3)/2; 1/sqrt(2)  1/sqrt(2)  1/sqrt(2) ]"  Multiplication=Matrix(K*u) (u vector)  SaturateOnIntegerOverflow=on  OutDataTypeStr=Inherit: Same as input  ParamDataTypeStr=Inherit: Same as input
  al_be_0 : Outport  VectorParamsAs1DForOutWhenUnconnected=off
  wires:
  abc/1 -> Gain3/1
  Gain3/1 -> Gain1/1
  Gain1/1 -> al_be_0/1

== system main_SEPETC/controller 2/primary 1/(P) abc to dq2/abc to Alpha-Beta-Zero ==
  abc : Inport  PortDimensions=3
  Gain1 : Gain  Gain=sqrt(2/3)  SaturateOnIntegerOverflow=on  OutDataTypeStr=Inherit: Same as input  ParamDataTypeStr=Inherit: Same as input
  Gain3 : Gain  Gain="[ 1   -1/2   -1/2; 0   sqrt(3)/2   -sqrt(3)/2; 1/sqrt(2)  1/sqrt(2)  1/sqrt(2) ]"  Multiplication=Matrix(K*u) (u vector)  SaturateOnIntegerOverflow=on  OutDataTypeStr=Inherit: Same as input  ParamDataTypeStr=Inherit: Same as input
  al_be_0 : Outport  VectorParamsAs1DForOutWhenUnconnected=off
  wires:
  abc/1 -> Gain3/1
  Gain3/1 -> Gain1/1
  Gain1/1 -> al_be_0/1

== system main_SEPETC/controller 3/primary 3/(P) abc to dq1/abc to Alpha-Beta-Zero ==
  abc : Inport  PortDimensions=3
  Gain1 : Gain  Gain=sqrt(2/3)  SaturateOnIntegerOverflow=on  OutDataTypeStr=Inherit: Same as input  ParamDataTypeStr=Inherit: Same as input
  Gain3 : Gain  Gain="[ 1   -1/2   -1/2; 0   sqrt(3)/2   -sqrt(3)/2; 1/sqrt(2)  1/sqrt(2)  1/sqrt(2) ]"  Multiplication=Matrix(K*u) (u vector)  SaturateOnIntegerOverflow=on  OutDataTypeStr=Inherit: Same as input  ParamDataTypeStr=Inherit: Same as input
  al_be_0 : Outport  VectorParamsAs1DForOutWhenUnconnected=off
  wires:
  abc/1 -> Gain3/1
  Gain3/1 -> Gain1/1
  Gain1/1 -> al_be_0/1

== system main_SEPETC/controller 3/primary 3/(P) abc to dq2/abc to Alpha-Beta-Zero ==
  abc : Inport  PortDimensions=3
  Gain1 : Gain  Gain=sqrt(2/3)  SaturateOnIntegerOverflow=on  OutDataTypeStr=Inherit: Same as input  ParamDataTypeStr=Inherit: Same as input
  Gain3 : Gain  Gain="[ 1   -1/2   -1/2; 0   sqrt(3)/2   -sqrt(3)/2; 1/sqrt(2)  1/sqrt(2)  1/sqrt(2) ]"  Multiplication=Matrix(K*u) (u vector)  SaturateOnIntegerOverflow=on  OutDataTypeStr=Inherit: Same as input  ParamDataTypeStr=Inherit: Same as input
  al_be_0 : Outport  VectorParamsAs1DForOutWhenUnconnected=off
  wires:
  abc/1 -> Gain3/1
  Gain3/1 -> Gain1/1
  Gain1/1 -> al_be_0/1

== system main_SEPETC/controller 4/primary 3/Subsystem1/(P) abc to dq1 ==
  abc : Inport  PortDimensions=3
  wt : Inport  Port=2  PortDimensions=1
  Alpha-Beta-Zero to dq0 : spsAlphaBetaZerotodq0Lib/Alpha-Beta-Zero to dq0  Alignment=90 degrees behind phase A axis
      settings: SourceProductBaseCode=PS
  abc to Alpha-Beta-Zero : Subsystem  AncestorBlock=powerlib_meascontrol/Transformations/abc to Alpha-Beta-Zero  DialogController=POWERSYS.PowerSysDialog  LoadFcn=sps_rtmsupport('LoadFcn', gcbh);  StartFcn=sps_rtmsupport('StartFcn', gcbh);  StopFcn=sps_rtmsupport('StopFcn', gcbh);  mask(abc to Alpha-Beta-Zero Transformation){}
      mask help: Perform a Clarke transformation from a three-phase (abc) signal to a alpha-beta-zero stationary reference frame.
      settings: CopyFcn=sps_rtmsupport('CopyFcn', gcbh);  DeleteFcn=sps_rtmsupport('DeleteFcn', gcbh);  UndoDeleteFcn=sps_rtmsupport('UndoDeleteFcn', gcbh);  ModelCloseFcn=sps_rtmsupport('ModelCloseFcn', gcbh);  PreSaveFcn=sps_rtmsupport('PreSaveFcn', gcbh);  PostSaveFcn=sps_rtmsupport('PostSaveFcn', gcbh);  NameChangeFcn=sps_rtmsupport('NameChangeFcn', gcbh);  PreCopyFcn=sps_rtmsupport('PreCopyFcn', gcbh);  OpenFcn=sps_rtmsupport('OpenFcn', gcbh, []);  CloseFcn=sps_rtmsupport('CloseFcn', gcbh);  PreDeleteFcn=sps_rtmsupport('PreDeleteFcn', gcbh);
      mask Help: helpview(psbhelp);
      mask Display:
      | plot([0 1], [0,1])
      | text(0.15,0.7,'abc')
      | text(0.55, 0.3,'\alpha\beta0','texmode','on')
  dq0 : Outport  VectorParamsAs1DForOutWhenUnconnected=off
  wires:
  wt/1 -> Alpha-Beta-Zero to dq0/2
  abc/1 -> abc to Alpha-Beta-Zero/1(abc)
  Alpha-Beta-Zero to dq0/1 -> dq0/1
  abc to Alpha-Beta-Zero/1(al_be_0) -> Alpha-Beta-Zero to dq0/1

== system main_SEPETC/controller 4/primary 3/Subsystem1/(P) abc to dq2 ==
  abc : Inport  PortDimensions=3
  wt : Inport  Port=2  PortDimensions=1
  Alpha-Beta-Zero to dq0 : spsAlphaBetaZerotodq0Lib/Alpha-Beta-Zero to dq0  Alignment=90 degrees behind phase A axis
      settings: SourceProductBaseCode=PS
  abc to Alpha-Beta-Zero : Subsystem  AncestorBlock=powerlib_meascontrol/Transformations/abc to Alpha-Beta-Zero  DialogController=POWERSYS.PowerSysDialog  LoadFcn=sps_rtmsupport('LoadFcn', gcbh);  StartFcn=sps_rtmsupport('StartFcn', gcbh);  StopFcn=sps_rtmsupport('StopFcn', gcbh);  mask(abc to Alpha-Beta-Zero Transformation){}
      mask help: Perform a Clarke transformation from a three-phase (abc) signal to a alpha-beta-zero stationary reference frame.
      settings: CopyFcn=sps_rtmsupport('CopyFcn', gcbh);  DeleteFcn=sps_rtmsupport('DeleteFcn', gcbh);  UndoDeleteFcn=sps_rtmsupport('UndoDeleteFcn', gcbh);  ModelCloseFcn=sps_rtmsupport('ModelCloseFcn', gcbh);  PreSaveFcn=sps_rtmsupport('PreSaveFcn', gcbh);  PostSaveFcn=sps_rtmsupport('PostSaveFcn', gcbh);  NameChangeFcn=sps_rtmsupport('NameChangeFcn', gcbh);  PreCopyFcn=sps_rtmsupport('PreCopyFcn', gcbh);  OpenFcn=sps_rtmsupport('OpenFcn', gcbh, []);  CloseFcn=sps_rtmsupport('CloseFcn', gcbh);  PreDeleteFcn=sps_rtmsupport('PreDeleteFcn', gcbh);
      mask Help: helpview(psbhelp);
      mask Display:
      | plot([0 1], [0,1])
      | text(0.15,0.7,'abc')
      | text(0.55, 0.3,'\alpha\beta0','texmode','on')
  dq0 : Outport  VectorParamsAs1DForOutWhenUnconnected=off
  wires:
  wt/1 -> Alpha-Beta-Zero to dq0/2
  abc/1 -> abc to Alpha-Beta-Zero/1(abc)
  Alpha-Beta-Zero to dq0/1 -> dq0/1
  abc to Alpha-Beta-Zero/1(al_be_0) -> Alpha-Beta-Zero to dq0/1

== system main_SEPETC/controller 4/primary 3/Subsystem1/(P) abc to dq1/abc to Alpha-Beta-Zero ==
  abc : Inport  PortDimensions=3
  Gain1 : Gain  Gain=sqrt(2/3)  SaturateOnIntegerOverflow=on  OutDataTypeStr=Inherit: Same as input  ParamDataTypeStr=Inherit: Same as input
  Gain3 : Gain  Gain="[ 1   -1/2   -1/2; 0   sqrt(3)/2   -sqrt(3)/2; 1/sqrt(2)  1/sqrt(2)  1/sqrt(2) ]"  Multiplication=Matrix(K*u) (u vector)  SaturateOnIntegerOverflow=on  OutDataTypeStr=Inherit: Same as input  ParamDataTypeStr=Inherit: Same as input
  al_be_0 : Outport  VectorParamsAs1DForOutWhenUnconnected=off
  wires:
  abc/1 -> Gain3/1
  Gain3/1 -> Gain1/1
  Gain1/1 -> al_be_0/1

== system main_SEPETC/controller 4/primary 3/Subsystem1/(P) abc to dq2/abc to Alpha-Beta-Zero ==
  abc : Inport  PortDimensions=3
  Gain1 : Gain  Gain=sqrt(2/3)  SaturateOnIntegerOverflow=on  OutDataTypeStr=Inherit: Same as input  ParamDataTypeStr=Inherit: Same as input
  Gain3 : Gain  Gain="[ 1   -1/2   -1/2; 0   sqrt(3)/2   -sqrt(3)/2; 1/sqrt(2)  1/sqrt(2)  1/sqrt(2) ]"  Multiplication=Matrix(K*u) (u vector)  SaturateOnIntegerOverflow=on  OutDataTypeStr=Inherit: Same as input  ParamDataTypeStr=Inherit: Same as input
  al_be_0 : Outport  VectorParamsAs1DForOutWhenUnconnected=off
  wires:
  abc/1 -> Gain3/1
  Gain3/1 -> Gain1/1
  Gain1/1 -> al_be_0/1

== matlab function main_SEPETC/line to phase1 ==
  data: u input; y output
function y = fcn(u)
xa=(2*u(1)+u(2))/3;
xc=-(2*u(2)+u(1))/3;
xb=-xa-xc;
y=[xa;xb;xc];

== matlab function main_SEPETC/line to phase2 ==
  data: u input; y output
function y = fcn(u)
xa=(2*u(1)+u(2))/3;
xc=-(2*u(2)+u(1))/3;
xb=-xa-xc;
y=[xa;xb;xc];

== matlab function main_SEPETC/line to phase3 ==
  data: u input; y output
function y = fcn(u)
xa=(2*u(1)+u(2))/3;
xc=-(2*u(2)+u(1))/3;
xb=-xa-xc;
y=[xa;xb;xc];

== matlab function main_SEPETC/line to phase ==
  data: u input; y output
function y = fcn(u)
xa=(2*u(1)+u(2))/3;
xc=-(2*u(2)+u(1))/3;
xb=-xa-xc;
y=[xa;xb;xc];
